simulink model "six_plus_six_AcmsteeringV09_main_1lf"  (R2014a)
settings: Solver=FixedStepDiscrete  StartTime=0.0  StopTime=10.0  FixedStep=0.0005  RelTol=1e-3
InitFcn:
  | Veh_Par_wxt
undefined symbols (not defined in the file or in its folder): acc_spdctl, ag_thr, B, bra_em, bra_pre_gz2, bra_pre_gz34, bra_pre_yd, brakepre_dem_data, brakeTrq_dem_data, bratrq_max, ecucoder_acal, eff_tran, ESP_switch, G, guzhang_lf, guzhang_lm, guzhang_lr, guzhang_rf, guzhang_rm, guzhang_rr, kd1, kd2, ki1, ki2, kp1, kp2, L, myFIS, premax, Radius, RC_switch, s_opt_yi, s_opt_zhuan, s_opt_zhuan_add, s_opt_zhuan_table, spd_map_mot, spd_spdctl, speed_thr_park, TCS_switch, tras_ratio, trq_map_mot, trqmax_yd, trqmax_zx, trqmaxneg, v_gain, v_table, v_thr_park, zhidong_bianmazhi, zhidong_down, zhidong_up, zhidong_youmen, zhuanxiang_bianmazhi, zhuanxiang_down, zhuanxiang_up, zhuanxiang_youmen
libraries: simulink x980, ec5744lib x59, fuzblock x2
(part 6 of 25)

== system six_plus_six_AcmsteeringV09_main_1lf/Data_input/BMS5/BMS5 ==
  input : Inport
  Enable : EnablePort
  BMS5_15s_InstanceDisPower_Ad : Sum
  BMS5_15s_InstanceDisPower_Convert : DataTypeConversion  OutDataTypeStr=uint32
  BMS5_15s_InstanceDisPower_F : Gain  Gain=0.01
  BMS5_15s_InstanceDisPower_L : simulink/Logic and Bit Operations/Bitwise Operator  logicop=AND  UseBitMask=on  BitMask=65535  BitMaskRealWorld=Stored Integer
  BMS5_15s_InstanceDisPower_O : Constant  Value=0  OutDataTypeStr=single
  BMS5_15s_InstanceDisPower_S : ArithShift
  BMS5_15s_InstanceDisPower_Sub : Subsystem
  BMS5_15s_InstanceDisPower_sat : Saturate  UpperLimit=655.35  LowerLimit=0
  BMS5_15s_InstanceDisPowercv : DataTypeConversion
  BMS5_15s_InstanceDisPowerinput4_Ad : Sum
  BMS5_15s_InstanceDisPowerinput4_C : Constant  Value=256
  BMS5_15s_InstanceDisPowerinput4_P : Product
  BMS5_ContDischargePower_Ad : Sum
  BMS5_ContDischargePower_Convert : DataTypeConversion  OutDataTypeStr=uint32
  BMS5_ContDischargePower_F : Gain  Gain=0.01
  BMS5_ContDischargePower_L : simulink/Logic and Bit Operations/Bitwise Operator  logicop=AND  UseBitMask=on  BitMask=65535  BitMaskRealWorld=Stored Integer
  BMS5_ContDischargePower_O : Constant  Value=0  OutDataTypeStr=single
  BMS5_ContDischargePower_S : ArithShift
  BMS5_ContDischargePower_Sub : Subsystem
  BMS5_ContDischargePower_sat : Saturate  UpperLimit=655.35  LowerLimit=0
  BMS5_ContDischargePowercv : DataTypeConversion
  BMS5_ContDischargePowerinput2_Ad : Sum
  BMS5_ContDischargePowerinput2_C : Constant  Value=256
  BMS5_ContDischargePowerinput2_P : Product
  BMS5_FailureLevel_Ad : Sum
  BMS5_FailureLevel_Convert : DataTypeConversion  OutDataTypeStr=uint32
  BMS5_FailureLevel_F : Gain
  BMS5_FailureLevel_L : simulink/Logic and Bit Operations/Bitwise Operator  logicop=AND  UseBitMask=on  BitMask=255  BitMaskRealWorld=Stored Integer
  BMS5_FailureLevel_O : Constant  Value=0  OutDataTypeStr=single
  BMS5_FailureLevel_S : ArithShift
  BMS5_FailureLevel_Sub : Subsystem
  BMS5_FailureLevel_sat : Saturate  UpperLimit=255  LowerLimit=0
  BMS5_FailureLevelcv : DataTypeConversion
  BMS5_FeedbackPower_Ad : Sum
  BMS5_FeedbackPower_Convert : DataTypeConversion  OutDataTypeStr=uint32
  BMS5_FeedbackPower_F : Gain  Gain=0.01
  BMS5_FeedbackPower_L : simulink/Logic and Bit Operations/Bitwise Operator  logicop=AND  UseBitMask=on  BitMask=65535  BitMaskRealWorld=Stored Integer
  BMS5_FeedbackPower_O : Constant  Value=0  OutDataTypeStr=single
  BMS5_FeedbackPower_S : ArithShift
  BMS5_FeedbackPower_Sub : Subsystem
  BMS5_FeedbackPower_sat : Saturate  UpperLimit=655.35  LowerLimit=0
  BMS5_FeedbackPowercv : DataTypeConversion
  BMS5_FeedbackPowerinput6_Ad : Sum
  BMS5_FeedbackPowerinput6_C : Constant  Value=256
  BMS5_FeedbackPowerinput6_P : Product
  BMS5_UpDownRequest_Ad : Sum
  BMS5_UpDownRequest_Convert : DataTypeConversion  OutDataTypeStr=uint32
  BMS5_UpDownRequest_F : Gain
  BMS5_UpDownRequest_L : simulink/Logic and Bit Operations/Bitwise Operator  logicop=AND  UseBitMask=on  BitMask=255  BitMaskRealWorld=Stored Integer
  BMS5_UpDownRequest_O : Constant  Value=0  OutDataTypeStr=single
  BMS5_UpDownRequest_S : ArithShift
  BMS5_UpDownRequest_Sub : Subsystem
  BMS5_UpDownRequest_sat : Saturate  UpperLimit=255  LowerLimit=0
  BMS5_UpDownRequestcv : DataTypeConversion
  Demux : Demux  Outputs=8
  BMS5_UpDownRequest_Out : Outport
  BMS5_FeedbackPower_Out : Outport  Port=2
  BMS5_FailureLevel_Out : Outport  Port=3
  BMS5_ContDischargePower_Out : Outport  Port=4
  BMS5_15s_InstanceDisPower_Out : Outport  Port=5
  wires:
  BMS5_UpDownRequest_F/1 -> BMS5_UpDownRequest_Ad/1
  BMS5_UpDownRequest_O/1 -> BMS5_UpDownRequest_Ad/2
  BMS5_UpDownRequest_Ad/1 -> BMS5_UpDownRequest_sat/1
  BMS5_UpDownRequest_sat/1 -> BMS5_UpDownRequest_Out/1
  Demux/8 -> BMS5_UpDownRequest_Sub/1(In1)
  BMS5_UpDownRequest_Sub/1(Out1) -> BMS5_UpDownRequest_Convert/1
  BMS5_UpDownRequest_Convert/1 -> BMS5_UpDownRequest_L/1
  BMS5_UpDownRequest_L/1 -> BMS5_UpDownRequest_S/1
  BMS5_UpDownRequest_S/1 -> BMS5_UpDownRequestcv/1
  BMS5_UpDownRequestcv/1 -> BMS5_UpDownRequest_F/1
  BMS5_FeedbackPower_F/1 -> BMS5_FeedbackPower_Ad/1
  BMS5_FeedbackPower_O/1 -> BMS5_FeedbackPower_Ad/2
  BMS5_FeedbackPower_Ad/1 -> BMS5_FeedbackPower_sat/1
  BMS5_FeedbackPower_sat/1 -> BMS5_FeedbackPower_Out/1
  Demux/6 -> BMS5_FeedbackPowerinput6_P/1
  BMS5_FeedbackPowerinput6_C/1 -> BMS5_FeedbackPowerinput6_P/2
  BMS5_FeedbackPowerinput6_P/1 -> BMS5_FeedbackPowerinput6_Ad/1
  Demux/7 -> BMS5_FeedbackPowerinput6_Ad/2
  BMS5_FeedbackPowerinput6_Ad/1 -> BMS5_FeedbackPower_Sub/1(In1)
  BMS5_FeedbackPower_Sub/1(Out1) -> BMS5_FeedbackPower_Convert/1
  BMS5_FeedbackPower_Convert/1 -> BMS5_FeedbackPower_L/1
  BMS5_FeedbackPower_L/1 -> BMS5_FeedbackPower_S/1
  BMS5_FeedbackPower_S/1 -> BMS5_FeedbackPowercv/1
  BMS5_FeedbackPowercv/1 -> BMS5_FeedbackPower_F/1
  BMS5_FailureLevel_F/1 -> BMS5_FailureLevel_Ad/1
  BMS5_FailureLevel_O/1 -> BMS5_FailureLevel_Ad/2
  BMS5_FailureLevel_Ad/1 -> BMS5_FailureLevel_sat/1
  BMS5_FailureLevel_sat/1 -> BMS5_FailureLevel_Out/1
  Demux/1 -> BMS5_FailureLevel_Sub/1(In1)
  BMS5_FailureLevel_Sub/1(Out1) -> BMS5_FailureLevel_Convert/1
  BMS5_FailureLevel_Convert/1 -> BMS5_FailureLevel_L/1
  BMS5_FailureLevel_L/1 -> BMS5_FailureLevel_S/1
  BMS5_FailureLevel_S/1 -> BMS5_FailureLevelcv/1
  BMS5_FailureLevelcv/1 -> BMS5_FailureLevel_F/1
  BMS5_ContDischargePower_F/1 -> BMS5_ContDischargePower_Ad/1
  BMS5_ContDischargePower_O/1 -> BMS5_ContDischargePower_Ad/2
  BMS5_ContDischargePower_Ad/1 -> BMS5_ContDischargePower_sat/1
  BMS5_ContDischargePower_sat/1 -> BMS5_ContDischargePower_Out/1
  Demux/2 -> BMS5_ContDischargePowerinput2_P/1
  BMS5_ContDischargePowerinput2_C/1 -> BMS5_ContDischargePowerinput2_P/2
  BMS5_ContDischargePowerinput2_P/1 -> BMS5_ContDischargePowerinput2_Ad/1
  Demux/3 -> BMS5_ContDischargePowerinput2_Ad/2
  BMS5_ContDischargePowerinput2_Ad/1 -> BMS5_ContDischargePower_Sub/1(In1)
  BMS5_ContDischargePower_Sub/1(Out1) -> BMS5_ContDischargePower_Convert/1
  BMS5_ContDischargePower_Convert/1 -> BMS5_ContDischargePower_L/1
  BMS5_ContDischargePower_L/1 -> BMS5_ContDischargePower_S/1
  BMS5_ContDischargePower_S/1 -> BMS5_ContDischargePowercv/1
  BMS5_ContDischargePowercv/1 -> BMS5_ContDischargePower_F/1
  BMS5_15s_InstanceDisPower_F/1 -> BMS5_15s_InstanceDisPower_Ad/1
  BMS5_15s_InstanceDisPower_O/1 -> BMS5_15s_InstanceDisPower_Ad/2
  BMS5_15s_InstanceDisPower_Ad/1 -> BMS5_15s_InstanceDisPower_sat/1
  BMS5_15s_InstanceDisPower_sat/1 -> BMS5_15s_InstanceDisPower_Out/1
  Demux/4 -> BMS5_15s_InstanceDisPowerinput4_P/1
  BMS5_15s_InstanceDisPowerinput4_C/1 -> BMS5_15s_InstanceDisPowerinput4_P/2
  BMS5_15s_InstanceDisPowerinput4_P/1 -> BMS5_15s_InstanceDisPowerinput4_Ad/1
  Demux/5 -> BMS5_15s_InstanceDisPowerinput4_Ad/2
  BMS5_15s_InstanceDisPowerinput4_Ad/1 -> BMS5_15s_InstanceDisPower_Sub/1(In1)
  BMS5_15s_InstanceDisPower_Sub/1(Out1) -> BMS5_15s_InstanceDisPower_Convert/1
  BMS5_15s_InstanceDisPower_Convert/1 -> BMS5_15s_InstanceDisPower_L/1
  BMS5_15s_InstanceDisPower_L/1 -> BMS5_15s_InstanceDisPower_S/1
  BMS5_15s_InstanceDisPower_S/1 -> BMS5_15s_InstanceDisPowercv/1
  BMS5_15s_InstanceDisPowercv/1 -> BMS5_15s_InstanceDisPower_F/1
  input/1 -> Demux/1

== system six_plus_six_AcmsteeringV09_main_1lf/Data_input/BMS5_1/BMS5 ==
  input : Inport
  Enable : EnablePort
  BMS5_15s_InstanceDisPower_Ad : Sum
  BMS5_15s_InstanceDisPower_Convert : DataTypeConversion  OutDataTypeStr=uint32
  BMS5_15s_InstanceDisPower_F : Gain  Gain=0.01
  BMS5_15s_InstanceDisPower_L : simulink/Logic and Bit Operations/Bitwise Operator  logicop=AND  UseBitMask=on  BitMask=65535  BitMaskRealWorld=Stored Integer
  BMS5_15s_InstanceDisPower_O : Constant  Value=0  OutDataTypeStr=single
  BMS5_15s_InstanceDisPower_S : ArithShift
  BMS5_15s_InstanceDisPower_Sub : Subsystem
  BMS5_15s_InstanceDisPower_sat : Saturate  UpperLimit=655.35  LowerLimit=0
  BMS5_15s_InstanceDisPowercv : DataTypeConversion
  BMS5_15s_InstanceDisPowerinput4_Ad : Sum
  BMS5_15s_InstanceDisPowerinput4_C : Constant  Value=256
  BMS5_15s_InstanceDisPowerinput4_P : Product
  BMS5_ContDischargePower_Ad : Sum
  BMS5_ContDischargePower_Convert : DataTypeConversion  OutDataTypeStr=uint32
  BMS5_ContDischargePower_F : Gain  Gain=0.01
  BMS5_ContDischargePower_L : simulink/Logic and Bit Operations/Bitwise Operator  logicop=AND  UseBitMask=on  BitMask=65535  BitMaskRealWorld=Stored Integer
  BMS5_ContDischargePower_O : Constant  Value=0  OutDataTypeStr=single
  BMS5_ContDischargePower_S : ArithShift
  BMS5_ContDischargePower_Sub : Subsystem
  BMS5_ContDischargePower_sat : Saturate  UpperLimit=655.35  LowerLimit=0
  BMS5_ContDischargePowercv : DataTypeConversion
  BMS5_ContDischargePowerinput2_Ad : Sum
  BMS5_ContDischargePowerinput2_C : Constant  Value=256
  BMS5_ContDischargePowerinput2_P : Product
  BMS5_FailureLevel_Ad : Sum
  BMS5_FailureLevel_Convert : DataTypeConversion  OutDataTypeStr=uint32
  BMS5_FailureLevel_F : Gain
  BMS5_FailureLevel_L : simulink/Logic and Bit Operations/Bitwise Operator  logicop=AND  UseBitMask=on  BitMask=255  BitMaskRealWorld=Stored Integer
  BMS5_FailureLevel_O : Constant  Value=0  OutDataTypeStr=single
  BMS5_FailureLevel_S : ArithShift
  BMS5_FailureLevel_Sub : Subsystem
  BMS5_FailureLevel_sat : Saturate  UpperLimit=255  LowerLimit=0
  BMS5_FailureLevelcv : DataTypeConversion
  BMS5_FeedbackPower_Ad : Sum
  BMS5_FeedbackPower_Convert : DataTypeConversion  OutDataTypeStr=uint32
  BMS5_FeedbackPower_F : Gain  Gain=0.01
  BMS5_FeedbackPower_L : simulink/Logic and Bit Operations/Bitwise Operator  logicop=AND  UseBitMask=on  BitMask=65535  BitMaskRealWorld=Stored Integer
  BMS5_FeedbackPower_O : Constant  Value=0  OutDataTypeStr=single
  BMS5_FeedbackPower_S : ArithShift
  BMS5_FeedbackPower_Sub : Subsystem
  BMS5_FeedbackPower_sat : Saturate  UpperLimit=655.35  LowerLimit=0
  BMS5_FeedbackPowercv : DataTypeConversion
  BMS5_FeedbackPowerinput6_Ad : Sum
  BMS5_FeedbackPowerinput6_C : Constant  Value=256
  BMS5_FeedbackPowerinput6_P : Product
  BMS5_UpDownRequest_Ad : Sum
  BMS5_UpDownRequest_Convert : DataTypeConversion  OutDataTypeStr=uint32
  BMS5_UpDownRequest_F : Gain
  BMS5_UpDownRequest_L : simulink/Logic and Bit Operations/Bitwise Operator  logicop=AND  UseBitMask=on  BitMask=255  BitMaskRealWorld=Stored Integer
  BMS5_UpDownRequest_O : Constant  Value=0  OutDataTypeStr=single
  BMS5_UpDownRequest_S : ArithShift
  BMS5_UpDownRequest_Sub : Subsystem
  BMS5_UpDownRequest_sat : Saturate  UpperLimit=255  LowerLimit=0
  BMS5_UpDownRequestcv : DataTypeConversion
  Demux : Demux  Outputs=8
  BMS5_UpDownRequest_Out : Outport
  BMS5_FeedbackPower_Out : Outport  Port=2
  BMS5_FailureLevel_Out : Outport  Port=3
  BMS5_ContDischargePower_Out : Outport  Port=4
  BMS5_15s_InstanceDisPower_Out : Outport  Port=5
  wires:
  BMS5_UpDownRequest_F/1 -> BMS5_UpDownRequest_Ad/1
  BMS5_UpDownRequest_O/1 -> BMS5_UpDownRequest_Ad/2
  BMS5_UpDownRequest_Ad/1 -> BMS5_UpDownRequest_sat/1
  BMS5_UpDownRequest_sat/1 -> BMS5_UpDownRequest_Out/1
  Demux/8 -> BMS5_UpDownRequest_Sub/1(In1)
  BMS5_UpDownRequest_Sub/1(Out1) -> BMS5_UpDownRequest_Convert/1
  BMS5_UpDownRequest_Convert/1 -> BMS5_UpDownRequest_L/1
  BMS5_UpDownRequest_L/1 -> BMS5_UpDownRequest_S/1
  BMS5_UpDownRequest_S/1 -> BMS5_UpDownRequestcv/1
  BMS5_UpDownRequestcv/1 -> BMS5_UpDownRequest_F/1
  BMS5_FeedbackPower_F/1 -> BMS5_FeedbackPower_Ad/1
  BMS5_FeedbackPower_O/1 -> BMS5_FeedbackPower_Ad/2
  BMS5_FeedbackPower_Ad/1 -> BMS5_FeedbackPower_sat/1
  BMS5_FeedbackPower_sat/1 -> BMS5_FeedbackPower_Out/1
  Demux/6 -> BMS5_FeedbackPowerinput6_P/1
  BMS5_FeedbackPowerinput6_C/1 -> BMS5_FeedbackPowerinput6_P/2
  BMS5_FeedbackPowerinput6_P/1 -> BMS5_FeedbackPowerinput6_Ad/1
  Demux/7 -> BMS5_FeedbackPowerinput6_Ad/2
  BMS5_FeedbackPowerinput6_Ad/1 -> BMS5_FeedbackPower_Sub/1(In1)
  BMS5_FeedbackPower_Sub/1(Out1) -> BMS5_FeedbackPower_Convert/1
  BMS5_FeedbackPower_Convert/1 -> BMS5_FeedbackPower_L/1
  BMS5_FeedbackPower_L/1 -> BMS5_FeedbackPower_S/1
  BMS5_FeedbackPower_S/1 -> BMS5_FeedbackPowercv/1
  BMS5_FeedbackPowercv/1 -> BMS5_FeedbackPower_F/1
  BMS5_FailureLevel_F/1 -> BMS5_FailureLevel_Ad/1
  BMS5_FailureLevel_O/1 -> BMS5_FailureLevel_Ad/2
  BMS5_FailureLevel_Ad/1 -> BMS5_FailureLevel_sat/1
  BMS5_FailureLevel_sat/1 -> BMS5_FailureLevel_Out/1
  Demux/1 -> BMS5_FailureLevel_Sub/1(In1)
  BMS5_FailureLevel_Sub/1(Out1) -> BMS5_FailureLevel_Convert/1
  BMS5_FailureLevel_Convert/1 -> BMS5_FailureLevel_L/1
  BMS5_FailureLevel_L/1 -> BMS5_FailureLevel_S/1
  BMS5_FailureLevel_S/1 -> BMS5_FailureLevelcv/1
  BMS5_FailureLevelcv/1 -> BMS5_FailureLevel_F/1
  BMS5_ContDischargePower_F/1 -> BMS5_ContDischargePower_Ad/1
  BMS5_ContDischargePower_O/1 -> BMS5_ContDischargePower_Ad/2
  BMS5_ContDischargePower_Ad/1 -> BMS5_ContDischargePower_sat/1
  BMS5_ContDischargePower_sat/1 -> BMS5_ContDischargePower_Out/1
  Demux/2 -> BMS5_ContDischargePowerinput2_P/1
  BMS5_ContDischargePowerinput2_C/1 -> BMS5_ContDischargePowerinput2_P/2
  BMS5_ContDischargePowerinput2_P/1 -> BMS5_ContDischargePowerinput2_Ad/1
  Demux/3 -> BMS5_ContDischargePowerinput2_Ad/2
  BMS5_ContDischargePowerinput2_Ad/1 -> BMS5_ContDischargePower_Sub/1(In1)
  BMS5_ContDischargePower_Sub/1(Out1) -> BMS5_ContDischargePower_Convert/1
  BMS5_ContDischargePower_Convert/1 -> BMS5_ContDischargePower_L/1
  BMS5_ContDischargePower_L/1 -> BMS5_ContDischargePower_S/1
  BMS5_ContDischargePower_S/1 -> BMS5_ContDischargePowercv/1
  BMS5_ContDischargePowercv/1 -> BMS5_ContDischargePower_F/1
  BMS5_15s_InstanceDisPower_F/1 -> BMS5_15s_InstanceDisPower_Ad/1
  BMS5_15s_InstanceDisPower_O/1 -> BMS5_15s_InstanceDisPower_Ad/2
  BMS5_15s_InstanceDisPower_Ad/1 -> BMS5_15s_InstanceDisPower_sat/1
  BMS5_15s_InstanceDisPower_sat/1 -> BMS5_15s_InstanceDisPower_Out/1
  Demux/4 -> BMS5_15s_InstanceDisPowerinput4_P/1
  BMS5_15s_InstanceDisPowerinput4_C/1 -> BMS5_15s_InstanceDisPowerinput4_P/2
  BMS5_15s_InstanceDisPowerinput4_P/1 -> BMS5_15s_InstanceDisPowerinput4_Ad/1
  Demux/5 -> BMS5_15s_InstanceDisPowerinput4_Ad/2
  BMS5_15s_InstanceDisPowerinput4_Ad/1 -> BMS5_15s_InstanceDisPower_Sub/1(In1)
  BMS5_15s_InstanceDisPower_Sub/1(Out1) -> BMS5_15s_InstanceDisPower_Convert/1
  BMS5_15s_InstanceDisPower_Convert/1 -> BMS5_15s_InstanceDisPower_L/1
  BMS5_15s_InstanceDisPower_L/1 -> BMS5_15s_InstanceDisPower_S/1
  BMS5_15s_InstanceDisPower_S/1 -> BMS5_15s_InstanceDisPowercv/1
  BMS5_15s_InstanceDisPowercv/1 -> BMS5_15s_InstanceDisPower_F/1
  input/1 -> Demux/1

== system six_plus_six_AcmsteeringV09_main_1lf/Data_input/BMS5_2/BMS5 ==
  input : Inport
  Enable : EnablePort
  BMS5_15s_InstanceDisPower_Ad : Sum
  BMS5_15s_InstanceDisPower_Convert : DataTypeConversion  OutDataTypeStr=uint32
  BMS5_15s_InstanceDisPower_F : Gain  Gain=0.01
  BMS5_15s_InstanceDisPower_L : simulink/Logic and Bit Operations/Bitwise Operator  logicop=AND  UseBitMask=on  BitMask=65535  BitMaskRealWorld=Stored Integer
  BMS5_15s_InstanceDisPower_O : Constant  Value=0  OutDataTypeStr=single
  BMS5_15s_InstanceDisPower_S : ArithShift
  BMS5_15s_InstanceDisPower_Sub : Subsystem
  BMS5_15s_InstanceDisPower_sat : Saturate  UpperLimit=655.35  LowerLimit=0
  BMS5_15s_InstanceDisPowercv : DataTypeConversion
  BMS5_15s_InstanceDisPowerinput4_Ad : Sum
  BMS5_15s_InstanceDisPowerinput4_C : Constant  Value=256
  BMS5_15s_InstanceDisPowerinput4_P : Product
  BMS5_ContDischargePower_Ad : Sum
  BMS5_ContDischargePower_Convert : DataTypeConversion  OutDataTypeStr=uint32
  BMS5_ContDischargePower_F : Gain  Gain=0.01
  BMS5_ContDischargePower_L : simulink/Logic and Bit Operations/Bitwise Operator  logicop=AND  UseBitMask=on  BitMask=65535  BitMaskRealWorld=Stored Integer
  BMS5_ContDischargePower_O : Constant  Value=0  OutDataTypeStr=single
  BMS5_ContDischargePower_S : ArithShift
  BMS5_ContDischargePower_Sub : Subsystem
  BMS5_ContDischargePower_sat : Saturate  UpperLimit=655.35  LowerLimit=0
  BMS5_ContDischargePowercv : DataTypeConversion
  BMS5_ContDischargePowerinput2_Ad : Sum
  BMS5_ContDischargePowerinput2_C : Constant  Value=256
  BMS5_ContDischargePowerinput2_P : Product
  BMS5_FailureLevel_Ad : Sum
  BMS5_FailureLevel_Convert : DataTypeConversion  OutDataTypeStr=uint32
  BMS5_FailureLevel_F : Gain
  BMS5_FailureLevel_L : simulink/Logic and Bit Operations/Bitwise Operator  logicop=AND  UseBitMask=on  BitMask=255  BitMaskRealWorld=Stored Integer
  BMS5_FailureLevel_O : Constant  Value=0  OutDataTypeStr=single
  BMS5_FailureLevel_S : ArithShift
  BMS5_FailureLevel_Sub : Subsystem
  BMS5_FailureLevel_sat : Saturate  UpperLimit=255  LowerLimit=0
  BMS5_FailureLevelcv : DataTypeConversion
  BMS5_FeedbackPower_Ad : Sum
  BMS5_FeedbackPower_Convert : DataTypeConversion  OutDataTypeStr=uint32
  BMS5_FeedbackPower_F : Gain  Gain=0.01
  BMS5_FeedbackPower_L : simulink/Logic and Bit Operations/Bitwise Operator  logicop=AND  UseBitMask=on  BitMask=65535  BitMaskRealWorld=Stored Integer
  BMS5_FeedbackPower_O : Constant  Value=0  OutDataTypeStr=single
  BMS5_FeedbackPower_S : ArithShift
  BMS5_FeedbackPower_Sub : Subsystem
  BMS5_FeedbackPower_sat : Saturate  UpperLimit=655.35  LowerLimit=0
  BMS5_FeedbackPowercv : DataTypeConversion
  BMS5_FeedbackPowerinput6_Ad : Sum
  BMS5_FeedbackPowerinput6_C : Constant  Value=256
  BMS5_FeedbackPowerinput6_P : Product
  BMS5_UpDownRequest_Ad : Sum
  BMS5_UpDownRequest_Convert : DataTypeConversion  OutDataTypeStr=uint32
  BMS5_UpDownRequest_F : Gain
  BMS5_UpDownRequest_L : simulink/Logic and Bit Operations/Bitwise Operator  logicop=AND  UseBitMask=on  BitMask=255  BitMaskRealWorld=Stored Integer
  BMS5_UpDownRequest_O : Constant  Value=0  OutDataTypeStr=single
  BMS5_UpDownRequest_S : ArithShift
  BMS5_UpDownRequest_Sub : Subsystem
  BMS5_UpDownRequest_sat : Saturate  UpperLimit=255  LowerLimit=0
  BMS5_UpDownRequestcv : DataTypeConversion
  Demux : Demux  Outputs=8
  BMS5_UpDownRequest_Out : Outport
  BMS5_FeedbackPower_Out : Outport  Port=2
  BMS5_FailureLevel_Out : Outport  Port=3
  BMS5_ContDischargePower_Out : Outport  Port=4
  BMS5_15s_InstanceDisPower_Out : Outport  Port=5
  wires:
  BMS5_UpDownRequest_F/1 -> BMS5_UpDownRequest_Ad/1
  BMS5_UpDownRequest_O/1 -> BMS5_UpDownRequest_Ad/2
  BMS5_UpDownRequest_Ad/1 -> BMS5_UpDownRequest_sat/1
  BMS5_UpDownRequest_sat/1 -> BMS5_UpDownRequest_Out/1
  Demux/8 -> BMS5_UpDownRequest_Sub/1(In1)
  BMS5_UpDownRequest_Sub/1(Out1) -> BMS5_UpDownRequest_Convert/1
  BMS5_UpDownRequest_Convert/1 -> BMS5_UpDownRequest_L/1
  BMS5_UpDownRequest_L/1 -> BMS5_UpDownRequest_S/1
  BMS5_UpDownRequest_S/1 -> BMS5_UpDownRequestcv/1
  BMS5_UpDownRequestcv/1 -> BMS5_UpDownRequest_F/1
  BMS5_FeedbackPower_F/1 -> BMS5_FeedbackPower_Ad/1
  BMS5_FeedbackPower_O/1 -> BMS5_FeedbackPower_Ad/2
  BMS5_FeedbackPower_Ad/1 -> BMS5_FeedbackPower_sat/1
  BMS5_FeedbackPower_sat/1 -> BMS5_FeedbackPower_Out/1
  Demux/6 -> BMS5_FeedbackPowerinput6_P/1
  BMS5_FeedbackPowerinput6_C/1 -> BMS5_FeedbackPowerinput6_P/2
  BMS5_FeedbackPowerinput6_P/1 -> BMS5_FeedbackPowerinput6_Ad/1
  Demux/7 -> BMS5_FeedbackPowerinput6_Ad/2
  BMS5_FeedbackPowerinput6_Ad/1 -> BMS5_FeedbackPower_Sub/1(In1)
  BMS5_FeedbackPower_Sub/1(Out1) -> BMS5_FeedbackPower_Convert/1
  BMS5_FeedbackPower_Convert/1 -> BMS5_FeedbackPower_L/1
  BMS5_FeedbackPower_L/1 -> BMS5_FeedbackPower_S/1
  BMS5_FeedbackPower_S/1 -> BMS5_FeedbackPowercv/1
  BMS5_FeedbackPowercv/1 -> BMS5_FeedbackPower_F/1
  BMS5_FailureLevel_F/1 -> BMS5_FailureLevel_Ad/1
  BMS5_FailureLevel_O/1 -> BMS5_FailureLevel_Ad/2
  BMS5_FailureLevel_Ad/1 -> BMS5_FailureLevel_sat/1
  BMS5_FailureLevel_sat/1 -> BMS5_FailureLevel_Out/1
  Demux/1 -> BMS5_FailureLevel_Sub/1(In1)
  BMS5_FailureLevel_Sub/1(Out1) -> BMS5_FailureLevel_Convert/1
  BMS5_FailureLevel_Convert/1 -> BMS5_FailureLevel_L/1
  BMS5_FailureLevel_L/1 -> BMS5_FailureLevel_S/1
  BMS5_FailureLevel_S/1 -> BMS5_FailureLevelcv/1
  BMS5_FailureLevelcv/1 -> BMS5_FailureLevel_F/1
  BMS5_ContDischargePower_F/1 -> BMS5_ContDischargePower_Ad/1
  BMS5_ContDischargePower_O/1 -> BMS5_ContDischargePower_Ad/2
  BMS5_ContDischargePower_Ad/1 -> BMS5_ContDischargePower_sat/1
  BMS5_ContDischargePower_sat/1 -> BMS5_ContDischargePower_Out/1
  Demux/2 -> BMS5_ContDischargePowerinput2_P/1
  BMS5_ContDischargePowerinput2_C/1 -> BMS5_ContDischargePowerinput2_P/2
  BMS5_ContDischargePowerinput2_P/1 -> BMS5_ContDischargePowerinput2_Ad/1
  Demux/3 -> BMS5_ContDischargePowerinput2_Ad/2
  BMS5_ContDischargePowerinput2_Ad/1 -> BMS5_ContDischargePower_Sub/1(In1)
  BMS5_ContDischargePower_Sub/1(Out1) -> BMS5_ContDischargePower_Convert/1
  BMS5_ContDischargePower_Convert/1 -> BMS5_ContDischargePower_L/1
  BMS5_ContDischargePower_L/1 -> BMS5_ContDischargePower_S/1
  BMS5_ContDischargePower_S/1 -> BMS5_ContDischargePowercv/1
  BMS5_ContDischargePowercv/1 -> BMS5_ContDischargePower_F/1
  BMS5_15s_InstanceDisPower_F/1 -> BMS5_15s_InstanceDisPower_Ad/1
  BMS5_15s_InstanceDisPower_O/1 -> BMS5_15s_InstanceDisPower_Ad/2
  BMS5_15s_InstanceDisPower_Ad/1 -> BMS5_15s_InstanceDisPower_sat/1
  BMS5_15s_InstanceDisPower_sat/1 -> BMS5_15s_InstanceDisPower_Out/1
  Demux/4 -> BMS5_15s_InstanceDisPowerinput4_P/1
  BMS5_15s_InstanceDisPowerinput4_C/1 -> BMS5_15s_InstanceDisPowerinput4_P/2
  BMS5_15s_InstanceDisPowerinput4_P/1 -> BMS5_15s_InstanceDisPowerinput4_Ad/1
  Demux/5 -> BMS5_15s_InstanceDisPowerinput4_Ad/2
  BMS5_15s_InstanceDisPowerinput4_Ad/1 -> BMS5_15s_InstanceDisPower_Sub/1(In1)
  BMS5_15s_InstanceDisPower_Sub/1(Out1) -> BMS5_15s_InstanceDisPower_Convert/1
  BMS5_15s_InstanceDisPower_Convert/1 -> BMS5_15s_InstanceDisPower_L/1
  BMS5_15s_InstanceDisPower_L/1 -> BMS5_15s_InstanceDisPower_S/1
  BMS5_15s_InstanceDisPower_S/1 -> BMS5_15s_InstanceDisPowercv/1
  BMS5_15s_InstanceDisPowercv/1 -> BMS5_15s_InstanceDisPower_F/1
  input/1 -> Demux/1

== system six_plus_six_AcmsteeringV09_main_1lf/Data_input/Enabled Subsystem/Subsystem ==
  CANTransmit : ec5744lib/RapidECU_U3/04CANCommunication/CANTransmit  canmodule=1  canbuffer=59  canmessageid=hex2dec('0000')  canmessagetype=Standard(11-bit ID)  datalength=2  sampletime=-1
  Constant2 : Constant  Value=hex2dec('00')  SampleTime=-1
  Constant3 : Constant  Value=hex2dec('01')  SampleTime=-1
  Data Type Conversion3 : DataTypeConversion
  Data Type Conversion8 : DataTypeConversion
  Mux : Mux  Inputs=2
  Terminator2 : Terminator
  wires:
  Mux/1 -> CANTransmit/1
  Constant3/1 -> Data Type Conversion3/1
  CANTransmit/1 -> Terminator2/1
  Data Type Conversion3/1 -> Mux/1
  Data Type Conversion8/1 -> Mux/2
  Constant2/1 -> Data Type Conversion8/1

== system six_plus_six_AcmsteeringV09_main_1lf/Data_input/MCU0/MCU0 ==
  input : Inport
  Enable : EnablePort
  Demux : Demux  Outputs=8
  MCU0_ControlMode_Ad : Sum
  MCU0_ControlMode_Convert : DataTypeConversion  OutDataTypeStr=uint32
  MCU0_ControlMode_F : Gain
  MCU0_ControlMode_L : simulink/Logic and Bit Operations/Bitwise Operator  logicop=AND  UseBitMask=on  BitMask=4  BitMaskRealWorld=Stored Integer
  MCU0_ControlMode_O : Constant  Value=0  OutDataTypeStr=single
  MCU0_ControlMode_S : ArithShift  BitShiftNumber=2
  MCU0_ControlMode_Sub : Subsystem
  MCU0_ControlMode_sat : Saturate  UpperLimit=1  LowerLimit=0
  MCU0_ControlModecv : DataTypeConversion
  MCU0_EmergShutDown_Ad : Sum
  MCU0_EmergShutDown_Convert : DataTypeConversion  OutDataTypeStr=uint32
  MCU0_EmergShutDown_F : Gain
  MCU0_EmergShutDown_L : simulink/Logic and Bit Operations/Bitwise Operator  logicop=AND  UseBitMask=on  BitMask=128  BitMaskRealWorld=Stored Integer
  MCU0_EmergShutDown_O : Constant  Value=0  OutDataTypeStr=single
  MCU0_EmergShutDown_S : ArithShift  BitShiftNumber=7
  MCU0_EmergShutDown_Sub : Subsystem
  MCU0_EmergShutDown_sat : Saturate  UpperLimit=1  LowerLimit=0
  MCU0_EmergShutDowncv : DataTypeConversion
  MCU0_GearStatus_Ad : Sum
  MCU0_GearStatus_Convert : DataTypeConversion  OutDataTypeStr=uint32
  MCU0_GearStatus_F : Gain
  MCU0_GearStatus_L : simulink/Logic and Bit Operations/Bitwise Operator  logicop=AND  UseBitMask=on  BitMask=24  BitMaskRealWorld=Stored Integer
  MCU0_GearStatus_O : Constant  Value=0  OutDataTypeStr=single
  MCU0_GearStatus_S : ArithShift  BitShiftNumber=3
  MCU0_GearStatus_Sub : Subsystem
  MCU0_GearStatus_sat : Saturate  UpperLimit=3  LowerLimit=0
  MCU0_GearStatuscv : DataTypeConversion
  MCU0_HighVol_Ad : Sum
  MCU0_HighVol_Convert : DataTypeConversion  OutDataTypeStr=uint32
  MCU0_HighVol_F : Gain
  MCU0_HighVol_L : simulink/Logic and Bit Operations/Bitwise Operator  logicop=AND  UseBitMask=on  BitMask=32  BitMaskRealWorld=Stored Integer
  MCU0_HighVol_O : Constant  Value=0  OutDataTypeStr=single
  MCU0_HighVol_S : ArithShift  BitShiftNumber=5
  MCU0_HighVol_Sub : Subsystem
  MCU0_HighVol_sat : Saturate  UpperLimit=1  LowerLimit=0
  MCU0_HighVolcv : DataTypeConversion
  MCU0_LiftCnt_Ad : Sum
  MCU0_LiftCnt_Convert : DataTypeConversion  OutDataTypeStr=uint32
  MCU0_LiftCnt_F : Gain
  MCU0_LiftCnt_L : simulink/Logic and Bit Operations/Bitwise Operator  logicop=AND  UseBitMask=on  BitMask=255  BitMaskRealWorld=Stored Integer
  MCU0_LiftCnt_O : Constant  Value=0  OutDataTypeStr=single
  MCU0_LiftCnt_S : ArithShift
  MCU0_LiftCnt_Sub : Subsystem
  MCU0_LiftCnt_sat : Saturate  UpperLimit=255  LowerLimit=0
  MCU0_LiftCntcv : DataTypeConversion
  MCU0_ShutDowAllow_Ad : Sum
  MCU0_ShutDowAllow_Convert : DataTypeConversion  OutDataTypeStr=uint32
  MCU0_ShutDowAllow_F : Gain
  MCU0_ShutDowAllow_L : simulink/Logic and Bit Operations/Bitwise Operator  logicop=AND  UseBitMask=on  BitMask=64  BitMaskRealWorld=Stored Integer
  MCU0_ShutDowAllow_O : Constant  Value=0  OutDataTypeStr=single
  MCU0_ShutDowAllow_S : ArithShift  BitShiftNumber=6
  MCU0_ShutDowAllow_Sub : Subsystem
  MCU0_ShutDowAllow_sat : Saturate  UpperLimit=1  LowerLimit=0
  MCU0_ShutDowAllowcv : DataTypeConversion
  MCU0_SpeedFdk_Ad : Sum
  MCU0_SpeedFdk_Convert : DataTypeConversion  OutDataTypeStr=uint32
  MCU0_SpeedFdk_F : Gain
  MCU0_SpeedFdk_L : simulink/Logic and Bit Operations/Bitwise Operator  logicop=AND  UseBitMask=on  BitMask=65535  BitMaskRealWorld=Stored Integer
  MCU0_SpeedFdk_O : Constant  Value=-10000  OutDataTypeStr=single
  MCU0_SpeedFdk_S : ArithShift
  MCU0_SpeedFdk_Sub : Subsystem
  MCU0_SpeedFdk_sat : Saturate  UpperLimit=10000  LowerLimit=-10000
  MCU0_SpeedFdkcv : DataTypeConversion
  MCU0_SpeedFdkinput2_Ad : Sum
  MCU0_SpeedFdkinput2_C : Constant  Value=256
  MCU0_SpeedFdkinput2_P : Product
  MCU0_TorqueFdk_Ad : Sum
  MCU0_TorqueFdk_Convert : DataTypeConversion  OutDataTypeStr=uint32
  MCU0_TorqueFdk_F : Gain  Gain=0.1
  MCU0_TorqueFdk_L : simulink/Logic and Bit Operations/Bitwise Operator  logicop=AND  UseBitMask=on  BitMask=65535  BitMaskRealWorld=Stored Integer
  MCU0_TorqueFdk_O : Constant  Value=-1000  OutDataTypeStr=single
  MCU0_TorqueFdk_S : ArithShift
  MCU0_TorqueFdk_Sub : Subsystem
  MCU0_TorqueFdk_sat : Saturate  UpperLimit=1000  LowerLimit=-1000
  MCU0_TorqueFdkcv : DataTypeConversion
  MCU0_TorqueFdkinput4_Ad : Sum
  MCU0_TorqueFdkinput4_C : Constant  Value=256
  MCU0_TorqueFdkinput4_P : Product
  MCU0_TorqueMax_Ad : Sum
  MCU0_TorqueMax_Convert : DataTypeConversion  OutDataTypeStr=uint32
  MCU0_TorqueMax_F : Gain  Gain=0.1
  MCU0_TorqueMax_L : simulink/Logic and Bit Operations/Bitwise Operator  logicop=AND  UseBitMask=on  BitMask=65535  BitMaskRealWorld=Stored Integer
  MCU0_TorqueMax_O : Constant  Value=-1000  OutDataTypeStr=single
  MCU0_TorqueMax_S : ArithShift
  MCU0_TorqueMax_Sub : Subsystem
  MCU0_TorqueMax_sat : Saturate  UpperLimit=1000  LowerLimit=-1000
  MCU0_TorqueMaxcv : DataTypeConversion
  MCU0_TorqueMaxinput6_Ad : Sum
  MCU0_TorqueMaxinput6_C : Constant  Value=256
  MCU0_TorqueMaxinput6_P : Product
  MCU0_WorkStatus_Ad : Sum
  MCU0_WorkStatus_Convert : DataTypeConversion  OutDataTypeStr=uint32
  MCU0_WorkStatus_F : Gain
  MCU0_WorkStatus_L : simulink/Logic and Bit Operations/Bitwise Operator  logicop=AND  UseBitMask=on  BitMask=3  BitMaskRealWorld=Stored Integer
  MCU0_WorkStatus_O : Constant  Value=0  OutDataTypeStr=single
  MCU0_WorkStatus_S : ArithShift
  MCU0_WorkStatus_Sub : Subsystem
  MCU0_WorkStatus_sat : Saturate  UpperLimit=3  LowerLimit=0
  MCU0_WorkStatuscv : DataTypeConversion
  MCU0_TorqueMax_Out : Outport
  MCU0_EmergShutDown_Out : Outport  Port=2
  MCU0_ShutDowAllow_Out : Outport  Port=3
  MCU0_HighVol_Out : Outport  Port=4
  MCU0_LiftCnt_Out : Outport  Port=5
  MCU0_TorqueFdk_Out : Outport  Port=6
  MCU0_SpeedFdk_Out : Outport  Port=7
  MCU0_GearStatus_Out : Outport  Port=8
  MCU0_ControlMode_Out : Outport  Port=9
  MCU0_WorkStatus_Out : Outport  Port=10
  wires:
  MCU0_TorqueMax_F/1 -> MCU0_TorqueMax_Ad/1
  MCU0_TorqueMax_O/1 -> MCU0_TorqueMax_Ad/2
  MCU0_TorqueMax_Ad/1 -> MCU0_TorqueMax_sat/1
  MCU0_TorqueMax_sat/1 -> MCU0_TorqueMax_Out/1
  Demux/6 -> MCU0_TorqueMaxinput6_P/1
  MCU0_TorqueMaxinput6_C/1 -> MCU0_TorqueMaxinput6_P/2
  MCU0_TorqueMaxinput6_P/1 -> MCU0_TorqueMaxinput6_Ad/1
  Demux/7 -> MCU0_TorqueMaxinput6_Ad/2
  MCU0_TorqueMaxinput6_Ad/1 -> MCU0_TorqueMax_Sub/1(In1)
  MCU0_TorqueMax_Sub/1(Out1) -> MCU0_TorqueMax_Convert/1
  MCU0_TorqueMax_Convert/1 -> MCU0_TorqueMax_L/1
  MCU0_TorqueMax_L/1 -> MCU0_TorqueMax_S/1
  MCU0_TorqueMax_S/1 -> MCU0_TorqueMaxcv/1
  MCU0_TorqueMaxcv/1 -> MCU0_TorqueMax_F/1
  MCU0_EmergShutDown_F/1 -> MCU0_EmergShutDown_Ad/1
  MCU0_EmergShutDown_O/1 -> MCU0_EmergShutDown_Ad/2
  MCU0_EmergShutDown_Ad/1 -> MCU0_EmergShutDown_sat/1
  MCU0_EmergShutDown_sat/1 -> MCU0_EmergShutDown_Out/1
  Demux/1 -> MCU0_ControlMode_Sub/1(In1), MCU0_WorkStatus_Sub/1(In1), MCU0_GearStatus_Sub/1(In1), MCU0_HighVol_Sub/1(In1), MCU0_ShutDowAllow_Sub/1(In1), MCU0_EmergShutDown_Sub/1(In1)
  MCU0_EmergShutDown_Sub/1(Out1) -> MCU0_EmergShutDown_Convert/1
  MCU0_EmergShutDown_Convert/1 -> MCU0_EmergShutDown_L/1
  MCU0_EmergShutDown_L/1 -> MCU0_EmergShutDown_S/1
  MCU0_EmergShutDown_S/1 -> MCU0_EmergShutDowncv/1
  MCU0_EmergShutDowncv/1 -> MCU0_EmergShutDown_F/1
  MCU0_ShutDowAllow_F/1 -> MCU0_ShutDowAllow_Ad/1
  MCU0_ShutDowAllow_O/1 -> MCU0_ShutDowAllow_Ad/2
  MCU0_ShutDowAllow_Ad/1 -> MCU0_ShutDowAllow_sat/1
  MCU0_ShutDowAllow_sat/1 -> MCU0_ShutDowAllow_Out/1
  MCU0_ShutDowAllow_Sub/1(Out1) -> MCU0_ShutDowAllow_Convert/1
  MCU0_ShutDowAllow_Convert/1 -> MCU0_ShutDowAllow_L/1
  MCU0_ShutDowAllow_L/1 -> MCU0_ShutDowAllow_S/1
  MCU0_ShutDowAllow_S/1 -> MCU0_ShutDowAllowcv/1
  MCU0_ShutDowAllowcv/1 -> MCU0_ShutDowAllow_F/1
  MCU0_HighVol_F/1 -> MCU0_HighVol_Ad/1
  MCU0_HighVol_O/1 -> MCU0_HighVol_Ad/2
  MCU0_HighVol_Ad/1 -> MCU0_HighVol_sat/1
  MCU0_HighVol_sat/1 -> MCU0_HighVol_Out/1
  MCU0_HighVol_Sub/1(Out1) -> MCU0_HighVol_Convert/1
  MCU0_HighVol_Convert/1 -> MCU0_HighVol_L/1
  MCU0_HighVol_L/1 -> MCU0_HighVol_S/1
  MCU0_HighVol_S/1 -> MCU0_HighVolcv/1
  MCU0_HighVolcv/1 -> MCU0_HighVol_F/1
  MCU0_LiftCnt_F/1 -> MCU0_LiftCnt_Ad/1
  MCU0_LiftCnt_O/1 -> MCU0_LiftCnt_Ad/2
  MCU0_LiftCnt_Ad/1 -> MCU0_LiftCnt_sat/1
  MCU0_LiftCnt_sat/1 -> MCU0_LiftCnt_Out/1
  Demux/8 -> MCU0_LiftCnt_Sub/1(In1)
  MCU0_LiftCnt_Sub/1(Out1) -> MCU0_LiftCnt_Convert/1
  MCU0_LiftCnt_Convert/1 -> MCU0_LiftCnt_L/1
  MCU0_LiftCnt_L/1 -> MCU0_LiftCnt_S/1
  MCU0_LiftCnt_S/1 -> MCU0_LiftCntcv/1
  MCU0_LiftCntcv/1 -> MCU0_LiftCnt_F/1
  MCU0_TorqueFdk_F/1 -> MCU0_TorqueFdk_Ad/1
  MCU0_TorqueFdk_O/1 -> MCU0_TorqueFdk_Ad/2
  MCU0_TorqueFdk_Ad/1 -> MCU0_TorqueFdk_sat/1
  MCU0_TorqueFdk_sat/1 -> MCU0_TorqueFdk_Out/1
  Demux/4 -> MCU0_TorqueFdkinput4_P/1
  MCU0_TorqueFdkinput4_C/1 -> MCU0_TorqueFdkinput4_P/2
  MCU0_TorqueFdkinput4_P/1 -> MCU0_TorqueFdkinput4_Ad/1
  Demux/5 -> MCU0_TorqueFdkinput4_Ad/2
  MCU0_TorqueFdkinput4_Ad/1 -> MCU0_TorqueFdk_Sub/1(In1)
  MCU0_TorqueFdk_Sub/1(Out1) -> MCU0_TorqueFdk_Convert/1
  MCU0_TorqueFdk_Convert/1 -> MCU0_TorqueFdk_L/1
  MCU0_TorqueFdk_L/1 -> MCU0_TorqueFdk_S/1
  MCU0_TorqueFdk_S/1 -> MCU0_TorqueFdkcv/1
  MCU0_TorqueFdkcv/1 -> MCU0_TorqueFdk_F/1
  MCU0_SpeedFdk_F/1 -> MCU0_SpeedFdk_Ad/1
  MCU0_SpeedFdk_O/1 -> MCU0_SpeedFdk_Ad/2
  MCU0_SpeedFdk_Ad/1 -> MCU0_SpeedFdk_sat/1
  MCU0_SpeedFdk_sat/1 -> MCU0_SpeedFdk_Out/1
  Demux/2 -> MCU0_SpeedFdkinput2_P/1
  MCU0_SpeedFdkinput2_C/1 -> MCU0_SpeedFdkinput2_P/2
  MCU0_SpeedFdkinput2_P/1 -> MCU0_SpeedFdkinput2_Ad/1
  Demux/3 -> MCU0_SpeedFdkinput2_Ad/2
  MCU0_SpeedFdkinput2_Ad/1 -> MCU0_SpeedFdk_Sub/1(In1)
  MCU0_SpeedFdk_Sub/1(Out1) -> MCU0_SpeedFdk_Convert/1
  MCU0_SpeedFdk_Convert/1 -> MCU0_SpeedFdk_L/1
  MCU0_SpeedFdk_L/1 -> MCU0_SpeedFdk_S/1
  MCU0_SpeedFdk_S/1 -> MCU0_SpeedFdkcv/1
  MCU0_SpeedFdkcv/1 -> MCU0_SpeedFdk_F/1
  MCU0_GearStatus_F/1 -> MCU0_GearStatus_Ad/1
  MCU0_GearStatus_O/1 -> MCU0_GearStatus_Ad/2
  MCU0_GearStatus_Ad/1 -> MCU0_GearStatus_sat/1
  MCU0_GearStatus_sat/1 -> MCU0_GearStatus_Out/1
  MCU0_GearStatus_Sub/1(Out1) -> MCU0_GearStatus_Convert/1
  MCU0_GearStatus_Convert/1 -> MCU0_GearStatus_L/1
  MCU0_GearStatus_L/1 -> MCU0_GearStatus_S/1
  MCU0_GearStatus_S/1 -> MCU0_GearStatuscv/1
  MCU0_GearStatuscv/1 -> MCU0_GearStatus_F/1
  MCU0_ControlMode_F/1 -> MCU0_ControlMode_Ad/1
  MCU0_ControlMode_O/1 -> MCU0_ControlMode_Ad/2
  MCU0_ControlMode_Ad/1 -> MCU0_ControlMode_sat/1
  MCU0_ControlMode_sat/1 -> MCU0_ControlMode_Out/1
  MCU0_ControlMode_Sub/1(Out1) -> MCU0_ControlMode_Convert/1
  MCU0_ControlMode_Convert/1 -> MCU0_ControlMode_L/1
  MCU0_ControlMode_L/1 -> MCU0_ControlMode_S/1
  MCU0_ControlMode_S/1 -> MCU0_ControlModecv/1
  MCU0_ControlModecv/1 -> MCU0_ControlMode_F/1
  MCU0_WorkStatus_F/1 -> MCU0_WorkStatus_Ad/1
  MCU0_WorkStatus_O/1 -> MCU0_WorkStatus_Ad/2
  MCU0_WorkStatus_Ad/1 -> MCU0_WorkStatus_sat/1
  MCU0_WorkStatus_sat/1 -> MCU0_WorkStatus_Out/1
  MCU0_WorkStatus_Sub/1(Out1) -> MCU0_WorkStatus_Convert/1
  MCU0_WorkStatus_Convert/1 -> MCU0_WorkStatus_L/1
  MCU0_WorkStatus_L/1 -> MCU0_WorkStatus_S/1
  MCU0_WorkStatus_S/1 -> MCU0_WorkStatuscv/1
  MCU0_WorkStatuscv/1 -> MCU0_WorkStatus_F/1
  input/1 -> Demux/1

== matlab function six_plus_six_AcmsteeringV09_main_1lf/MainControl/mode_control/forward/forward/Drive/左右侧电机分配及功率限制/MATLAB Function ==
  data: trqlim_l input; trq_dem_l output; trq_dem_r output; trq_dem_l1 input; trqlim_r input; trq_dem_r1 input; delta_T_dem input
function [trq_dem_l,trq_dem_r] = fcn(trqlim_l,trq_dem_l1,trqlim_r,trq_dem_r1,delta_T_dem)
%#codegen
if trq_dem_l1==trqlim_l
    trq_dem_l=single(trq_dem_l1);
    trq_dem_r=single(trq_dem_l1+delta_T_dem);%这时候加的是负值
elseif trq_dem_r1==trqlim_r
    trq_dem_l=single(trq_dem_r1-delta_T_dem);
    trq_dem_r=single(trq_dem_r1);
    
else
    trq_dem_l=single(trq_dem_l1);
    trq_dem_r=single(trq_dem_r1);
end
% trq_dem_l=single(max(0,trq_dem_l));%限一下最小值，不要小于0
% trq_dem_r=single(max(0,trq_dem_r));
trq_dem_l=single(max(-trqlim_l,trq_dem_l));%小转向半径下，内侧履带是可能输出负转矩的，从地面吸收功率，给外侧，所以不能限到0，限到最大电机外特性负值
trq_dem_r=single(max(-trqlim_r,trq_dem_r));
end

== matlab function six_plus_six_AcmsteeringV09_main_1lf/MainControl/mode_control/forward/forward/Drive/驱动防滑控制TCS/直行TCS/直行/HeartBeat3 ==
  data: life_pre input; life output
function life = fcn(life_pre)
%#codegen
life=single(life_pre+1);
if life>255
    life=single(0);
end
end

== matlab function six_plus_six_AcmsteeringV09_main_1lf/MainControl/mode_control/forward/forward/Drive/驱动防滑控制TCS/直行TCS/直行/HeartBeat4 ==
  data: life_pre input; life output
function life = fcn(life_pre)
%#codegen
life=single(life_pre+1);
if life>255
    life=single(0);
end
end

== matlab function six_plus_six_AcmsteeringV09_main_1lf/MainControl/mode_control/forward/forward/Drive/驱动防滑控制TCS/直行TCS/直行/HeartBeat1 ==
  data: life_pre input; life output
function life = fcn(life_pre)
%#codegen
life=single(life_pre+1);
if life>255
    life=single(0);
end
end

== matlab function six_plus_six_AcmsteeringV09_main_1lf/MainControl/mode_control/forward/forward/Drive/驱动防滑控制TCS/直行TCS/直行/HeartBeat5 ==
  data: life_pre input; life output
function life = fcn(life_pre)
%#codegen
life=single(life_pre+1);
if life>255
    life=single(0);
end
end

== matlab function six_plus_six_AcmsteeringV09_main_1lf/MainControl/mode_control/forward/forward/Brake/HeartBeat2 ==
  data: life_pre input; life output
function life = fcn(life_pre)
%#codegen
life=single(life_pre+1);
if life>255
    life=single(0);
end
end

== matlab function six_plus_six_AcmsteeringV09_main_1lf/MainControl/mode_control/forward/forward/Brake/HeartBeat3 ==
  data: life_pre input; life output
function life = fcn(life_pre)
%#codegen
life=single(life_pre+1);
if life>255
    life=single(0);
end
end

== matlab function six_plus_six_AcmsteeringV09_main_1lf/MainControl/mode_control/forward/forward/Brake/HeartBeat4 ==
  data: life_pre input; life output
function life = fcn(life_pre)
%#codegen
life=single(life_pre+1);
if life>255
    life=single(0);
end
end

== matlab function six_plus_six_AcmsteeringV09_main_1lf/MainControl/mode_control/forward/forward/Brake/HeartBeat1 ==
  data: life_pre input; life output
function life = fcn(life_pre)
%#codegen
life=single(life_pre+1);
if life>255
    life=single(0);
end
end

== matlab function six_plus_six_AcmsteeringV09_main_1lf/MainControl/mode_control/forward/forward/Brake/HeartBeat5 ==
  data: life_pre input; life output
function life = fcn(life_pre)
%#codegen
life=single(life_pre+1);
if life>255
    life=single(0);
end
end

== matlab function six_plus_six_AcmsteeringV09_main_1lf/Data_input/3/Enabled Subsystem/MATLAB Function1 ==
  data: current_in input; current_out output
function current_out = motec_current(current_in)
    if current_in>32768
        current_out=current_in-65535;
    else
        current_out=current_in;
    end
end

== matlab function six_plus_six_AcmsteeringV09_main_1lf/MainControl/mode_control/neutral/neutral/HeartBeat1 ==
  data: life_pre input; life output
function life = fcn(life_pre)
%#codegen
life=single(life_pre+1);
if life>255
    life=single(0);
end
end

== matlab function six_plus_six_AcmsteeringV09_main_1lf/MainControl/mode_control/neutral/neutral/HeartBeat2 ==
  data: life_pre input; life output
function life = fcn(life_pre)
%#codegen
life=single(life_pre+1);
if life>255
    life=single(0);
end
end

== matlab function six_plus_six_AcmsteeringV09_main_1lf/MainControl/mode_control/backward/backward/Brake/HeartBeat ==
  data: life_pre input; life output
function life = fcn(life_pre)
%#codegen
life=single(life_pre+1);
if life>255
    life=single(0);
end
end

== matlab function six_plus_six_AcmsteeringV09_main_1lf/MainControl/mode_control/backward/backward/Brake/HeartBeat2 ==
  data: life_pre input; life output
function life = fcn(life_pre)
%#codegen
life=single(life_pre+1);
if life>255
    life=single(0);
end
end

== matlab function six_plus_six_AcmsteeringV09_main_1lf/MainControl/mode_control/backward/backward/Brake/HeartBeat4 ==
  data: life_pre input; life output
function life = fcn(life_pre)
%#codegen
life=single(life_pre+1);
if life>255
    life=single(0);
end
end

== matlab function six_plus_six_AcmsteeringV09_main_1lf/MainControl/mode_control/backward/backward/Brake/Switch Case Action Subsystem/MATLAB Function5 ==
  data: bratrq_dem_lf input; bratrq_dem_lm input; bratrq_dem_lr input; bratrq_dem_rf input; bratrq_dem_rm input; bratrq_dem_rr input; pwr_chg_bat input; bratrq_mot_lf output; bratrq_mot_lm output; pwr_chg_bat1 input; pwr_chg_bat2 input; trqlimL_dig_lf input; bratrq_mot_lr output; bratrq_mot_rf output; bratrq_mot_rm output; bratrq_mot_rr output; trqlimL_dig_lm input; trqlimL_dig_lr input; trqlimL_dig_rf input; trqlimL_dig_rm input; trqlimL_dig_rr input; speed_act_lf input; speed_act_lm input; speed_act_lr input; speed_act_rf input; speed_act_rm input; speed_act_rr input; trqlim_map_lf input; brapre_out_l output; brapre_out_r output; trqlim_map_lm input; trqlim_map_lr input; trqlim_map_rf input; trqlim_map_rm input; trqlim_map_rr input; tras_ratio input; guzhang_lf input; guzhang_lm input; guzhang_lr input; guzhang_rf input; guzhang_rm input; guzhang_rr input
function [bratrq_mot_lf,bratrq_mot_lm,bratrq_mot_lr,bratrq_mot_rf,bratrq_mot_rm,bratrq_mot_rr,brapre_out_l,brapre_out_r] = fcn(bratrq_dem_lf,bratrq_dem_lm,bratrq_dem_lr,bratrq_dem_rf,bratrq_dem_rm,bratrq_dem_rr,pwr_chg_bat,pwr_chg_bat1,pwr_chg_bat2,trqlimL_dig_lf,trqlimL_dig_lm,trqlimL_dig_lr,trqlimL_dig_rf,trqlimL_dig_rm,trqlimL_dig_rr,speed_act_lf,speed_act_lm,speed_act_lr,speed_act_rf,speed_act_rm,speed_act_rr,trqlim_map_lf,trqlim_map_lm,trqlim_map_lr,trqlim_map_rf,trqlim_map_rm,trqlim_map_rr,tras_ratio,guzhang_lf,guzhang_lm,guzhang_lr,guzhang_rf,guzhang_rm,guzhang_rr)
%#codegen pid模块在外面做，里面进行十六种情况的判断，先看一下效果，不能再修改。前轴单独控制，后轴低选控制

bratrq_mot_lf1=single(bratrq_dem_lf/tras_ratio);
bratrq_mot_lf2=single(9549*(pwr_chg_bat/2)/speed_act_lf);
bratrq_mot_lf=single(min(trqlimL_dig_lf,min(bratrq_mot_lf1,bratrq_mot_lf2)));

bratrq_mot_lm1=single(bratrq_dem_lm/tras_ratio);
bratrq_mot_lm2=single(9549*(pwr_chg_bat1/2)/speed_act_lm);
bratrq_mot_lm=single(min(trqlimL_dig_lm,min(bratrq_mot_lm1,bratrq_mot_lm2)));

bratrq_mot_lr1=single(bratrq_dem_lr/tras_ratio);
bratrq_mot_lr2=single(9549*(pwr_chg_bat2/2)/speed_act_lr);
bratrq_mot_lr=single(min(trqlimL_dig_lr,min(bratrq_mot_lr1,bratrq_mot_lr2)));
 
bratrq_mot_rf1=single(bratrq_dem_rf/tras_ratio);
bratrq_mot_rf2=single(9549*(pwr_chg_bat/2)/speed_act_rf);
bratrq_mot_rf=single(min(trqlimL_dig_rf,min(bratrq_mot_rf1,bratrq_mot_rf2)));

bratrq_mot_rm1=single(bratrq_dem_rm/tras_ratio);
bratrq_mot_rm2=single(9549*(pwr_chg_bat1/2)/speed_act_rm);
bratrq_mot_rm=single(min(trqlimL_dig_rm,min(bratrq_mot_rm1,bratrq_mot_rm2)));

bratrq_mot_rr1=single(bratrq_dem_rr/tras_ratio);
bratrq_mot_rr2=single(9549*(pwr_chg_bat2/2)/speed_act_rr);
bratrq_mot_rr=single(min(trqlimL_dig_rr,min(bratrq_mot_rr1,bratrq_mot_rr2)));

brapre_out_l=single(((bratrq_dem_lf+bratrq_dem_lm+bratrq_dem_lr)-(bratrq_mot_lf+bratrq_mot_lm+bratrq_mot_lr)*tras_ratio)/3/150);
brapre_out_r=single(((bratrq_dem_rf+bratrq_dem_rm+bratrq_dem_rr)-(bratrq_mot_rf+bratrq_mot_rm+bratrq_mot_rr)*tras_ratio)/3/150);







bratrq_mot_lf=single(min(bratrq_mot_lf,trqlim_map_lf));%限一下最大值在外特性内，最小值大于0
bratrq_mot_lf=single(max(bratrq_mot_lf,0));
bratrq_mot_lr=single(min(bratrq_mot_lr,trqlim_map_lr));
bratrq_mot_lr=single(max(bratrq_mot_lr,0));
bratrq_mot_rf=single(min(bratrq_mot_rf,trqlim_map_rf));
bratrq_mot_rf=single(max(bratrq_mot_rf,0));
bratrq_mot_rr=single(min(bratrq_mot_rr,trqlim_map_rr));
bratrq_mot_rr=single(max(bratrq_mot_rr,0));

% brapre_out_l=brapre_out_l;
% brapre_out_r=brapre_out_r;
brapre_out_l=single(brapre_out_l*150/125);%第二辆车的制动压力与制动力的关系调整一下。
brapre_out_r=single(brapre_out_r*150/125);

if guzhang_lf==1
    bratrq_mot_lf=single(0);
end
if guzhang_lm==1
    bratrq_mot_lm=single(0);
end
if guzhang_lr==1
    bratrq_mot_lr=single(0);
end
if guzhang_rf==1
    bratrq_mot_rf=single(0);
end
if guzhang_rm==1
    bratrq_mot_rm=single(0);
end
if guzhang_rr==1
    bratrq_mot_rr=single(0);
end

end

== matlab function six_plus_six_AcmsteeringV09_main_1lf/MainControl/mode_control/center_steer/center_steer/HeartBeat4 ==
  data: life_pre input; life output
function life = fcn(life_pre)
%#codegen
life=single(life_pre+1);
if life>255
    life=single(0);
end
end

== matlab function six_plus_six_AcmsteeringV09_main_1lf/MainControl/mode_control/emergency_stop/emergency_stop/HeartBeat2 ==
  data: life_pre input; life output
function life = fcn(life_pre)
%#codegen
life=single(life_pre+1);
if life>255
    life=single(0);
end
end

== matlab function six_plus_six_AcmsteeringV09_main_1lf/Data_input/181/Enabled
Subsystem/MATLAB Function1 ==
  data: current_in input; current_out output
function current_out = motec_current(current_in)
    if current_in>32768
        current_out=current_in-65535;
    else
        current_out=current_in;
    end
end

== matlab function six_plus_six_AcmsteeringV09_main_1lf/MainControl/mode_switch/mode_switch ==
  data: brake_emerg input; park input; mode_dem_out output int8; acc_dem input; steer_dem input; brake_dem input; center input; MCU0_SpeedFdk input; MCU0_1SpeedFdk input; MCU0_2SpeedFdk input; MCU0_3SpeedFdk input; MCU0_4SpeedFdk input; MCU0_5SpeedFdk input; speed_thr_park input; mode_dem_out_pre input
 function mode_dem_out = fcn(brake_emerg,park,acc_dem,steer_dem,brake_dem,center,MCU0_SpeedFdk,MCU0_1SpeedFdk,MCU0_2SpeedFdk,MCU0_3SpeedFdk,MCU0_4SpeedFdk,MCU0_5SpeedFdk,speed_thr_park,mode_dem_out_pre)
%#codegen
mode_dem_out=int8(mode_dem_out_pre);

if park==1  && MCU0_SpeedFdk<=speed_thr_park && MCU0_1SpeedFdk<=speed_thr_park && MCU0_2SpeedFdk<=speed_thr_park && MCU0_3SpeedFdk<=speed_thr_park  && MCU0_4SpeedFdk<=speed_thr_park  && MCU0_5SpeedFdk<=speed_thr_park && brake_emerg==0
    mode_dem_out=int8(0);
elseif acc_dem>0 && MCU0_SpeedFdk>=0 && MCU0_1SpeedFdk>=0 && MCU0_2SpeedFdk>=0 && MCU0_3SpeedFdk>=0  && MCU0_4SpeedFdk>=0  && MCU0_5SpeedFdk>=0 && brake_emerg==0  && park==0  && center==0
    mode_dem_out=int8(1);
elseif acc_dem==0 && brake_emerg==0  && park==0  && center==0
    mode_dem_out=int8(2);
elseif acc_dem<0 && MCU0_SpeedFdk>=0 && MCU0_1SpeedFdk>=0 && MCU0_2SpeedFdk>=0 && MCU0_3SpeedFdk>=0  && MCU0_4SpeedFdk>=0  && MCU0_5SpeedFdk>=0 && brake_emerg==0  && park==0  && center==0
    mode_dem_out=int8(3);
elseif center==1  && brake_emerg==0  && park==0        
    mode_dem_out=int8(1);
elseif brake_emerg==1
    mode_dem_out=int8(5);   
% else
%     mode_dem_out=int8(5);
end



end

== matlab function six_plus_six_AcmsteeringV09_main_1lf/Data_input/7/Enabled Subsystem/MATLAB Function1 ==
  data: data1 input; y output; data2 input; data3 input; data4 input
function y = fcn(data1,data2,data3,data4)
%#codegen
y1=data4*256^3+data3*256^2+data2*256+data1;
y=typecast(uint32(y1),'single');
end
% y = u;

== matlab function six_plus_six_AcmsteeringV09_main_1lf/Data_input/10/Enabled Subsystem/MATLAB Function1 ==
  data: data1 input; y output; data2 input; data3 input; data4 input
function y = fcn(data1,data2,data3,data4)
%#codegen
y1=data4*256^3+data3*256^2+data2*256+data1;
y=typecast(uint32(y1),'single');
end
% y = u;

== matlab function six_plus_six_AcmsteeringV09_main_1lf/MainControl/mode_control/Park/park/HeartBeat2 ==
  data: life_pre input; life output
function life = fcn(life_pre)
%#codegen
life=single(life_pre+1);
if life>255
    life=single(0);
end
end
